simulink model "chap11_6sim"  (Simulink 6.3)
settings: Solver=ode45  StartTime=0.0  StopTime=10  RelTol=1e-3
values from neighbouring files (symbols this model uses):
  b = 1    [chap11_4int.m]    (also in chap11_6int.m = 0.5)
  f1 = (b+kd*kv)    (= 12.5)    [chap11_6int.m]
  f2 = J    (= 2)    [chap11_6int.m]
  J = 1.0    (= 1)    [chap11_1plant.m]    (also in chap11_2.m = 0.6; chap11_3plant.m = 0.6; chap11_4int.m = 2; chap11_6int.m = 2)
  kd = 6    [chap11_4int.m]    (also in chap11_5int.m; chap11_6int.m)
  kp = 15    [chap11_6int.m]
  kv = 2.0    (= 2)    [chap11_2plant.m]    (also in chap11_3plant.m; chap11_4int.m; chap11_5int.m; chap11_6int.m)
settings Model: LastModifiedBy=Administrator  ExtModeTrigMode=oneshot  ExtModeArmWhenConnect=off  StrictBusMsg=None
settings DataIOCC: LimitDataPoints=off
settings OptimizationCC: BlockReduction=off  BooleanDataType=off
settings DebuggingCC: SolverPrmCheckMsg=none
settings HardwareCC: TargetUnknown=on

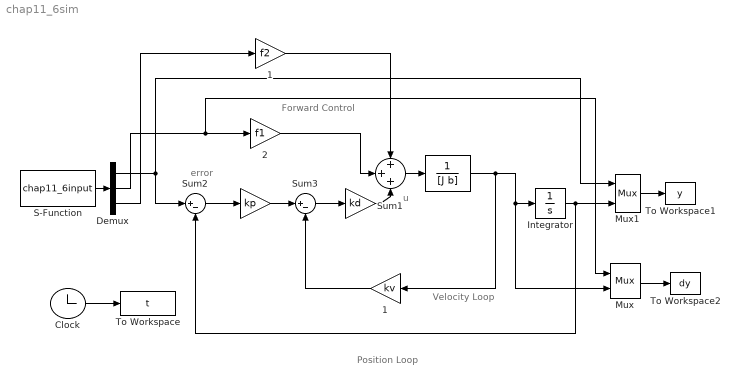
== system chap11_6sim ==
  note: u
  note: Position Loop
  note: Velocity Loop
  note: Forward Control
  note: error
  " " : TransferFcn  Denominator=[J b]
  "  " : Gain  Gain=kd  SaturateOnIntegerOverflow=on
  "   " : Gain  Gain=kp  SaturateOnIntegerOverflow=on
  "   1" : Gain  Orientation=left  Gain=kv  SaturateOnIntegerOverflow=on
  "   2" : Gain  Gain=f1
  "  1" : Gain  Gain=f2
  Clock : Clock
      settings: Decimation=10
  Demux : Demux  Outputs=3
  Integrator : Integrator
  Mux : Mux  Inputs=2
  Mux1 : Mux  Inputs=2
  S-Function : S-Function  FunctionName=chap11_6input
  Sum1 : Sum  Inputs=+++  InputSameDT=on
  Sum2 : Sum  Inputs=|+-  SaturateOnIntegerOverflow=on  InputSameDT=on
  Sum3 : Sum  Inputs=|+-  SaturateOnIntegerOverflow=on  InputSameDT=on
  To Workspace : ToWorkspace  VariableName=t  SampleTime=-1  SaveFormat=Array
  To Workspace1 : ToWorkspace  VariableName=y  SampleTime=-1  SaveFormat=Array
  To Workspace2 : ToWorkspace  VariableName=dy  SampleTime=-1  SaveFormat=Array
  wires:
  "  1"/1 -> Sum1/1
  Sum2/1 -> "   "/1
  "  "/1 -> Sum1/3
  "   1"/1 -> Sum3/2
  Sum3/1 -> "  "/1
  "   "/1 -> Sum3/1
  "   2"/1 -> Sum1/2
  Sum1/1 -> " "/1
  Mux/1 -> To Workspace2/1
  Mux1/1 -> To Workspace1/1
  Integrator/1 -> Sum2/2, Mux1/2
  " "/1 -> Integrator/1, Mux/2, "   1"/1
  Clock/1 -> To Workspace/1
  S-Function/1 -> Demux/1
  Demux/1 -> Sum2/1, Mux1/1
  Demux/2 -> "   2"/1, Mux/1
  Demux/3 -> "  1"/1
